simulink model "fir_filter"  (R2023a)
settings: Solver=VariableStepAuto  StartTime=0.0  StopTime=10.0  RelTol=1e-3
settings Model: Creator=metti  LastModifiedBy=metti

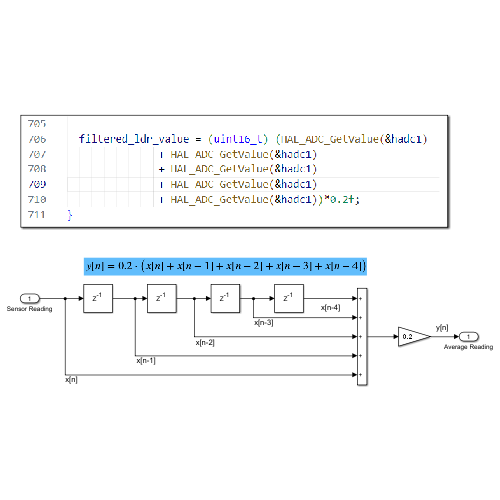
[thumbnail: Simulink's stored preview of the top-level diagram]
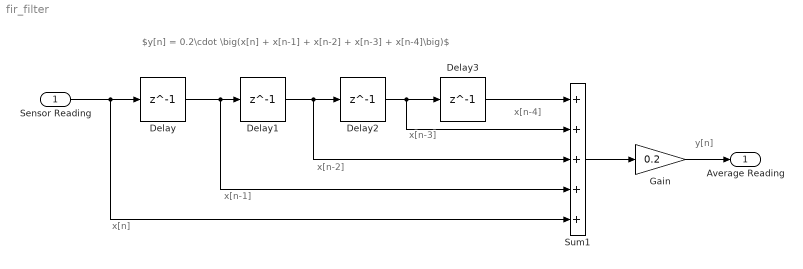
== system fir_filter ==
  note: $y[n] = 0.2\cdot \big(x[n] + x[n-1] + x[n-2] + x[n-3] + x[n-4]\big)$
  note: y[n]
  note: x[n-4]
  note: x[n-3]
  note: x[n-2]
  note: x[n-1]
  note: x[n]
  Sensor Reading : Inport
  Delay{,1..3} (4 alike) : Delay  DelayLength=1
  Gain : Gain  Gain=0.2
  Sum1 : Sum  Inputs=+++++
  Average Reading : Outport
  wires:
  Sensor Reading/1 -> Sum1/5, Delay/1
  Delay/1 -> Delay1/1, Sum1/4
  Delay1/1 -> Delay2/1, Sum1/3
  Sum1/1 -> Gain/1
  Gain/1 -> Average Reading/1
  Delay2/1 -> Sum1/2, Delay3/1
  Delay3/1 -> Sum1/1
